simulink model "PIOModel15a"  (R2015a)
settings: Solver=ode23  SolverMode=SingleTasking  StartTime=0.0  StopTime=Tsim  RelTol=1e-3
values from neighbouring files (symbols this model uses):
  A = [-1 1;0 -2]    [PIO_init.m]
  B = [0;1]    [PIO_init.m]
  C = eye(2)    [PIO_init.m]
  X_0 = zeros(2,1)    [PIO_init.m]
undefined symbols (not defined in the file or in its folder): Ap, Li, Lp, Xhat_0, xY_0
settings Model: CovMetricSettings=dwe  CovHtmlReporting=off  covSaveCumulativeToWorkspaceVar=off  CovSaveSingleToWorkspaceVar=off  CovExternalEMLEnable=on  Creator=samnazari  LastModifiedBy=sam
settings DataIOCC: LimitDataPoints=off  SaveFormat=Dataset
settings DebuggingCC: SFUnexpectedBacktrackingDiag=error  SFNoUnconditionalDefaultTransitionDiag=error
settings HardwareCC: ProdBitPerPointer=64  ProdLargestAtomicFloat=Float  ProdIntDivRoundTo=Zero  ProdEndianess=LittleEndian  ProdHWDeviceType=Specified
settings ModelReferenceCC: PropagateSignalLabelsOutOfModel=on
settings GRTTargetCC: TargetLangStandard=C99 (ISO)  GeneratePreprocessorConditionals=Use local settings

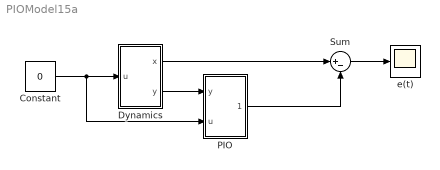
== system PIOModel15a ==
  Constant : Constant  Value=0
  Dynamics : Subsystem
  PIO : Subsystem
  Sum : Sum  Inputs=|+-
  "e(t) " : Scope
      settings: TimeRange=auto  MaxDataPoints=5000  SaveToWorkspace=off  SaveName=ScopeData  YMin=-0.21537  YMax=0.61639  SampleTime=-1
  wires:
  Dynamics/2(y) -> PIO/1(y)
  Constant/1 -> PIO/2(u), Dynamics/1(u)
  PIO/1(xHat) -> Sum/2
  Dynamics/1(x) -> Sum/1
  Sum/1 -> "e(t) "/1

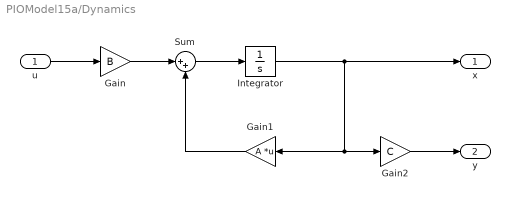
== system PIOModel15a/Dynamics ==
  u : Inport
  Gain : Gain  Gain=B
  Gain1 : Gain  Gain=A  Multiplication=Matrix(K*u)
  Gain2 : Gain  Gain=C
  Integrator : Integrator  InitialCondition=X_0
  Sum : Sum  Inputs=|++
  x : Outport
  y : Outport  Port=2
  wires:
  Gain/1 -> Sum/1
  Integrator/1 -> x/1, Gain2/1, Gain1/1
  Gain1/1 -> Sum/2
  Sum/1 -> Integrator/1
  u/1 -> Gain/1
  Gain2/1 -> y/1

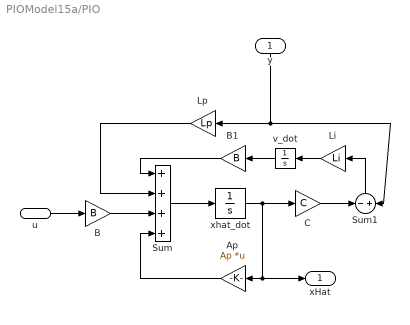
== system PIOModel15a/PIO ==
  y : Inport
  u : Inport  Port=2
  Ap : Gain  Gain=Ap  Multiplication=Matrix(K*u)
  B : Gain  Gain=B
  B1 : Gain  Gain=B
  C : Gain  Gain=C
  Li : Gain  Gain=Li
  Lp : Gain  Gain=Lp
  Sum : Sum  Inputs=++++
  Sum1 : Sum  Inputs=-+
  v_dot : Integrator  InitialCondition=xY_0
  xhat_dot : Integrator  InitialCondition=Xhat_0
  xHat : Outport
  wires:
  B1/1 -> Sum/1
  u/1 -> B/1
  y/1 -> Lp/1, Sum1/2
  Ap/1 -> Sum/4
  Sum/1 -> xhat_dot/1
  Sum1/1 -> Li/1
  C/1 -> Sum1/1
  B/1 -> Sum/3
  Lp/1 -> Sum/2
  xhat_dot/1 -> C/1, xHat/1, Ap/1
  Li/1 -> v_dot/1
  v_dot/1 -> B1/1
